simulink library "COMH"  (R2016a)
settings: Solver=ode45  StartTime=0.0  StopTime=10.0  RelTol=1e-3
undefined symbols (not defined in the file): ROB_ERRVAL, ROB_LENG, ROB_NONE, ROB_NORTH, SAMPLE_TIME
settings Model: Creator=oelkawok  LastModifiedBy=omaro
settings DataIOCC: LimitDataPoints=on
settings DebuggingCC: AllowSymbolicDim=off

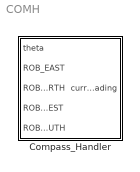
== system COMH ==
  Compass_Handler : Subsystem

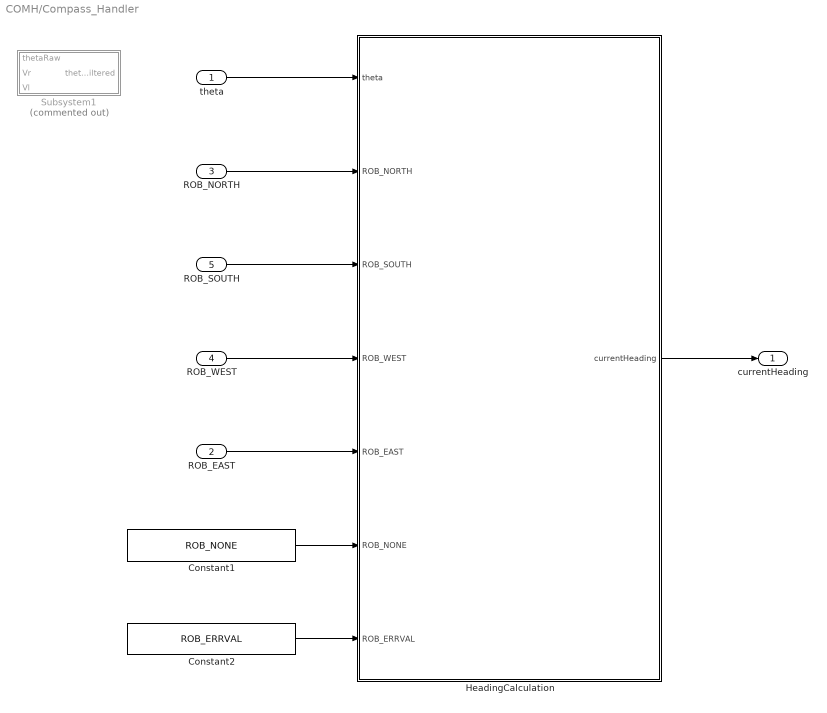
== system COMH/Compass_Handler ==
  theta : Inport
  ROB_EAST : Inport  Port=2  PortDimensions=1
  ROB_NORTH : Inport  Port=3  PortDimensions=1
  ROB_WEST : Inport  Port=4  PortDimensions=1
  ROB_SOUTH : Inport  Port=5  PortDimensions=1
  Constant1 : Constant  Value=ROB_NONE
  Constant2 : Constant  Value=ROB_ERRVAL
  HeadingCalculation : Stateflow chart  TreatAsAtomicUnit=on
  Subsystem1 : Subsystem  Commented=on
  currentHeading : Outport
  wires:
  HeadingCalculation/1(currentHeading) -> currentHeading/1
  theta/1 -> HeadingCalculation/1(theta)
  ROB_NORTH/1 -> HeadingCalculation/2(ROB_NORTH)
  ROB_SOUTH/1 -> HeadingCalculation/3(ROB_SOUTH)
  ROB_WEST/1 -> HeadingCalculation/4(ROB_WEST)
  ROB_EAST/1 -> HeadingCalculation/5(ROB_EAST)
  Constant1/1 -> HeadingCalculation/6(ROB_NONE)
  Constant2/1 -> HeadingCalculation/7(ROB_ERRVAL)

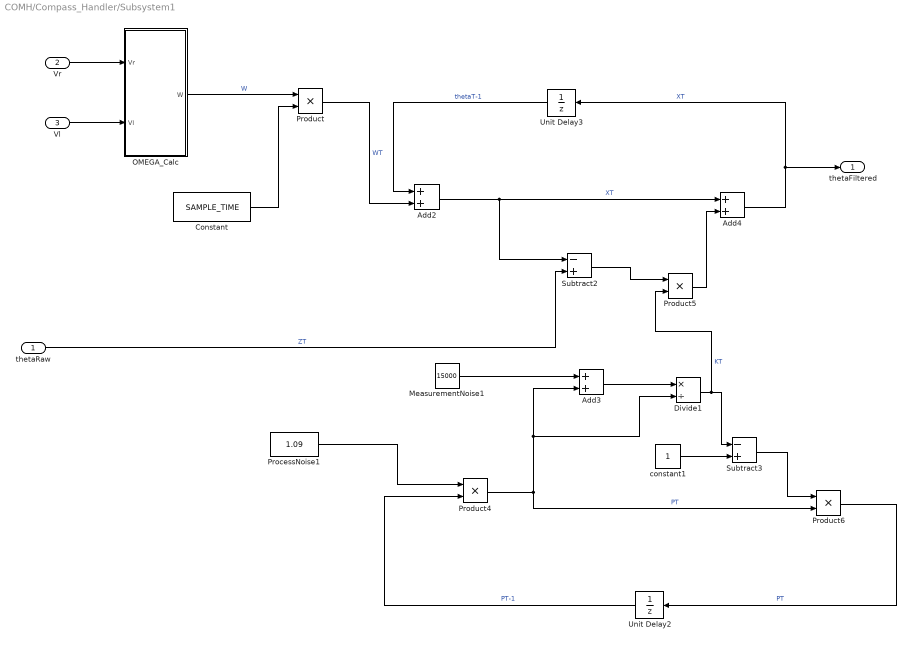
== system COMH/Compass_Handler/Subsystem1 ==
  thetaRaw : Inport
  Vr : Inport  Port=2
  Vl : Inport  Port=3
  Add2 : Sum
  Add3 : Sum
  Add4 : Sum
  Constant : Constant  Value=SAMPLE_TIME
  Divide1 : Product  Inputs=*/
  MeasurementNoise1 : Constant  Value=15000
  OMEGA_Calc : Subsystem
  ProcessNoise1 : Constant  Value=1.09
  Product{,4..6} (4 alike) : Product
  Subtract2 : Sum  Inputs=-+
  Subtract3 : Sum  Inputs=-+
  Unit Delay2 : UnitDelay  InitialCondition=1  SampleTime=-1
  Unit Delay3 : UnitDelay  InitialCondition=ROB_NORTH*100  SampleTime=-1
  constant1 : Constant
  thetaFiltered : Outport
  wires:
  Add4/1 -> Unit Delay3/1, thetaFiltered/1  "XT"
  Product5/1 -> Add4/2
  Product6/1 -> Unit Delay2/1  "PT"
  Subtract3/1 -> Product6/1
  constant1/1 -> Subtract3/2
  Subtract2/1 -> Product5/1
  Add2/1 -> Add4/1, Subtract2/1  "XT"
  Divide1/1 -> Product5/2, Subtract3/1  "KT"
  Add3/1 -> Divide1/1
  MeasurementNoise1/1 -> Add3/1
  Product4/1 -> Add3/2, Divide1/2, Product6/2  "PT"
  Unit Delay2/1 -> Product4/2  "PT-1"
  ProcessNoise1/1 -> Product4/1
  Unit Delay3/1 -> Add2/1  "thetaT-1"
  Product/1 -> Add2/2  "WT"
  thetaRaw/1 -> Subtract2/2  "ZT"
  OMEGA_Calc/1(W) -> Product/1  "W"
  Constant/1 -> Product/2
  Vr/1 -> OMEGA_Calc/1(Vr)
  Vl/1 -> OMEGA_Calc/2(Vl)

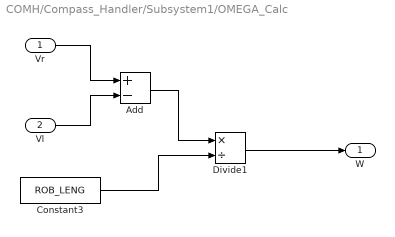
== system COMH/Compass_Handler/Subsystem1/OMEGA_Calc ==
  Vr : Inport
  Vl : Inport  Port=2
  Add : Sum  Inputs=+-
  Constant3 : Constant  Value=ROB_LENG
  Divide1 : Product  Inputs=*/
  W : Outport
  wires:
  Add/1 -> Divide1/1
  Divide1/1 -> W/1
  Constant3/1 -> Divide1/2
  Vr/1 -> Add/1
  Vl/1 -> Add/2

== stateflow chart COMH/Compass_Handler/HeadingCalculation ==
  state initializeDirection
    entry:
    offset = theta;
  state Calc
    entry:
    theta_OUT = theta;
    //remove for now - offset
  state CalcHeading
    (default) -> (junction 2)
    (junction 2) -> (junction 3) [order 1] : [(theta_OUT <= 270 + ROB_ERRVAL) && (theta_OUT >= 270 - ROB_ERRVAL)]//NORTH
    (junction 2) -> (junction 4) [order 2]
    (junction 3) -> (junction 17) : {currentHeading = ROB_NORTH;}
    (junction 4) -> (junction 5) [order 1] : [(theta_OUT <= 90 + ROB_ERRVAL) && (theta_OUT >= 90 - ROB_ERRVAL)]//SOUTH
    (junction 4) -> (junction 6) [order 2]
    (junction 5) -> (junction 16) : {currentHeading = ROB_SOUTH;}
    (junction 6) -> (junction 7) [order 1] : [(theta_OUT <= 0 + ROB_ERRVAL) || (theta_OUT >= 360 - ROB_ERRVAL)]//EAST
    (junction 6) -> (junction 8) [order 2]
    (junction 7) -> (junction 15) : {currentHeading = ROB_EAST;}
    (junction 8) -> (junction 9) [order 1] : [(theta_OUT <= 180 + ROB_ERRVAL) && (theta_OUT >= 180 - ROB_ERRVAL)]//WEST
    (junction 8) -> (junction 12) [order 2] : {currentHeading = ROB_NONE;}
    (junction 9) -> (junction 14) : {currentHeading = ROB_WEST;}
    (junction 14) -> (junction 12)
    (junction 15) -> (junction 14)
    (junction 16) -> (junction 15)
    (junction 17) -> (junction 16)
    (junction 12) -> (junction 18)
  Calc -> CalcHeading [order 3]
  (default) -> initializeDirection
  initializeDirection -> Calc
  Calc -> (junction 54) [order 1] : [theta_OUT < 0]
  (junction 54) -> CalcHeading : /theta_OUT = theta_OUT + 360;
  CalcHeading -> Calc : [hasChanged(theta)]
  Calc -> (junction 57) [order 2] : [theta_OUT < ROB_ERRVAL]
  (junction 57) -> CalcHeading : /theta_OUT = ROB_ERRVAL;
  data: theta input; ROB_NORTH input; ROB_SOUTH input; ROB_WEST input; ROB_EAST input; ROB_NONE input; ROB_ERRVAL input; theta_OUT local int16; currentHeading output uint16; offset local int16
